simulink model "ES248A_MotAgArbn"  (R2013b)
settings: Solver=FixedStepDiscrete  StartTime=0.0  StopTime=2  FixedStep=0.00005  RelTol=1e-3
undefined symbols (not defined in the file): MAXSTALL_CNT_U08, sigbuilder_block
libraries: simulink x6
settings Model: ModifiedHistory=Rev 008: Updated model to Matlab 2013B, added comments to show requirement linkage  Creator=nz3zln  LastModifiedBy=TZBSJD
settings DataIOCC: SignalLoggingSaveFormat=ModelDataLogs
settings OptimizationCC: InlineParams=on  ExpressionDepthLimit=2147483647
settings DebuggingCC: MultiTaskDSMMsg=none  FcnCallInpInsideContextMsg=UseLocalSettings  StateNameClashWarn=warning
settings GRTTargetCC: CombineOutputUpdateFcns=off  GRTInterface=on

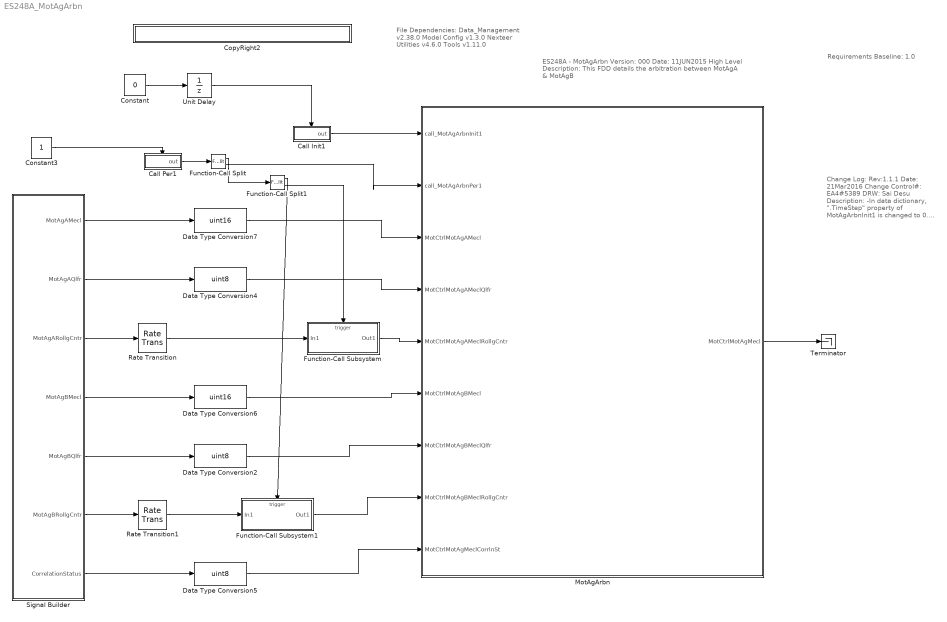
== system ES248A_MotAgArbn ==
  note: ES248A - MotAgArbn
      |
      | Version: 000
      | Date: 11JUN2015
      |
      | High Level Description:
      | This FDD details the arbitration between MotAgA & MotAgB
  note: Change Log:
      | Rev:1.1.1
      | Date: 21Mar2016
      | Change Control#: EA4#5389
      | DRW: Sai Desu
      | Description:
      |  -In data dictionary, ".TimeStep"
      | property of  MotAgArbnInit1 is
      | changed to 0.
      | -In data dictionary, ".Context"
      | property of  MotAgArbnper1 is
      | changed to NonRte.
      |
      | Rev: 1.1.0
      | Date: 13OCT2015
      | Change Control #: EA4#1850
      | DRW: Muragesh Asundi
      | Description:
      | - Init function added
      |
      | Rev: 1.0.0
      | Date: 11JUN2015
      | Change Control #: ICR-TBD
      | DRW: J. Erlenbeck
      | Description:
      | - Initial Release
  note: File Dependencies:
      | Data_Management v2.38.0
      | Model Config v1.3.0
      | Nexteer Utilities v4.6.0
      | Tools v1.11.0
  note: Requirements Baseline: 1.0
  Call Init1 : Subsystem  TreatAsAtomicUnit=on
  Call Per1 : Subsystem  TreatAsAtomicUnit=on
  Constant : Constant  Value=0  OutDataTypeStr=uint8
  Constant3 : Constant  OutDataTypeStr=int8
  CopyRight2 : Subsystem  Description=|  mask(Copyright Information){none=on}
      | Copyright info block.                                               
      |                                                                     
      | Place copyright information at the top of every subsystem in design.
      mask prompts: none "No parameters"
      mask help: Place copyright information at the top of every subsystem in design.
      mask Display:
      | NxtrConf = 'Nexteer Confidential';
      | 
      | sys = bdroot; %handle for the current model ("system")
      | first = get_param(sys,'Created');
      | first = first(end-3:end);  %year is last four digits
      | 
      | last = get_param(sys,'LastModifiedDate');
      | if isempty(last)
      |     last = datestr(now,'yyyy');
      | else
      |     last = last(end-3:end);
      | end
      | 
      | if strcmp(first,last)
      |     fprintf('%s -- Copyright %s Nexteer',NxtrConf,first)
      | else
      |     fprintf('%s -- %s%s- %s Nexteer',NxtrConf,char(169),first,last)
      | end
  Data Type Conversion2 : DataTypeConversion  OutDataTypeStr=uint8  RndMeth=Nearest
  Data Type Conversion4 : DataTypeConversion  OutDataTypeStr=uint8  RndMeth=Nearest
  Data Type Conversion5 : DataTypeConversion  OutDataTypeStr=uint8  RndMeth=Nearest
  Data Type Conversion6 : DataTypeConversion  OutDataTypeStr=uint16  RndMeth=Nearest
  Data Type Conversion7 : DataTypeConversion  OutDataTypeStr=uint16  RndMeth=Nearest
  Function-Call Split : FunctionCallSplit
  Function-Call Split1 : FunctionCallSplit
  Function-Call Subsystem : Subsystem  TreatAsAtomicUnit=on
  Function-Call Subsystem1 : Subsystem  TreatAsAtomicUnit=on
  MotAgArbn : Subsystem
  Rate Transition : RateTransition
  Rate Transition1 : RateTransition
  Signal Builder : Subsystem  Tag=STV Subsys  LoadFcn=sigbuilder_block('load');  StartFcn=sigbuilder_block('start');  StopFcn=sigbuilder_block('stop');  ClipboardFcn=sigbuilder_block('clipboard');  mask(Sigbuilder block){}
      mask help: Simulink:masks:SigbuilderBlock_MD
      mask init:
      | if ~strcmp(get_param(bdroot(gcbh),'SimulationStatus'),'stopped') tuvar = sigbuilder_block('maskInit'); end
      settings: CopyFcn=sigbuilder_block('copy');  DeleteFcn=sigbuilder_block('delete');  ModelCloseFcn=sigbuilder_block('modelClose');  PreSaveFcn=sigbuilder_block('preSave');  PauseFcn=sigbuilder_block('pause');  ContinueFcn=sigbuilder_block('continue');  NameChangeFcn=sigbuilder_block('namechange');  OpenFcn=sigbuilder_block('open',[130.345 51.5172 968.276 555.517 ]);  CloseFcn=sigbuilder_block('close');
      mask Display: plot(0, 0, 100, 100,[2, 2, 32, 32, 2], [68, 8, 8, 68, 68],[32, 2], [38, 38], [32, 19, 2],[53, 60, 44], [32, 17, 17, 2],[16, 16, 31, 31]);txt = getActiveGroup(gcbh);text(2, 100, txt,'verticalAlignment', 'top');
  Terminator : Terminator
  Unit Delay : UnitDelay  InitialCondition=1  SampleTime=-1
  wires:
  Constant3/1 -> Call Per1/Enable
  Call Per1/1(out) -> Function-Call Split/1
  Signal Builder/5(MotAgBQlfr) -> Data Type Conversion2/1
  Signal Builder/4(MotAgBMecl) -> Data Type Conversion6/1
  Signal Builder/3(MotAgARollgCntr) -> Rate Transition/1
  Signal Builder/7(CorrelationStatus) -> Data Type Conversion5/1
  Signal Builder/2(MotAgAQlfr) -> Data Type Conversion4/1
  Signal Builder/1(MotAgAMecl) -> Data Type Conversion7/1
  Data Type Conversion4/1 -> MotAgArbn/4(MotCtrlMotAgAMeclQlfr)
  Data Type Conversion2/1 -> MotAgArbn/7(MotCtrlMotAgBMeclQlfr)
  Data Type Conversion5/1 -> MotAgArbn/9(MotCtrlMotAgMeclCorrlnSt)
  Data Type Conversion6/1 -> MotAgArbn/6(MotCtrlMotAgBMecl)
  Data Type Conversion7/1 -> MotAgArbn/3(MotCtrlMotAgAMecl)
  Function-Call Subsystem/1(Out1) -> MotAgArbn/5(MotCtrlMotAgAMeclRollgCntr)
  Rate Transition/1 -> Function-Call Subsystem/1(In1)
  Signal Builder/6(MotAgBRollgCntr) -> Rate Transition1/1
  Rate Transition1/1 -> Function-Call Subsystem1/1(In1)
  Function-Call Subsystem1/1(Out1) -> MotAgArbn/8(MotCtrlMotAgBMeclRollgCntr)
  Function-Call Split/2 -> MotAgArbn/2(call_MotAgArbnPer1)
  Function-Call Split/1 -> Function-Call Split1/1
  Function-Call Split1/2 -> Function-Call Subsystem/Trigger
  Function-Call Split1/1 -> Function-Call Subsystem1/Trigger
  Call Init1/1(out) -> MotAgArbn/1(call_MotAgArbnInit1)
  Constant/1 -> Unit Delay/1
  Unit Delay/1 -> Call Init1/Enable
  MotAgArbn/1("MotCtrlMotAgMecl ") -> Terminator/1

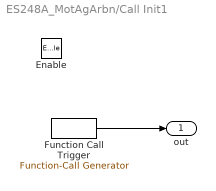
== system ES248A_MotAgArbn/Call Init1 ==
  Enable : EnablePort
  Function Call Trigger : simulink/Ports & Subsystems/Function-Call Generator  RequirementInfo={} %GIDa_03d3be70_2a53_4f3d_90ce_b287f92bdd04  sample_time=0.0005  numberOfIterations=1
  out : Outport
  wires:
  Function Call Trigger/1 -> out/1

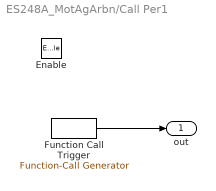
== system ES248A_MotAgArbn/Call Per1 ==
  Enable : EnablePort
  Function Call Trigger : simulink/Ports & Subsystems/Function-Call Generator  RequirementInfo={} %GIDa_6dd05ab1_f91b_4d7a_a0ec_1170d213fa7b  sample_time=0.0005  numberOfIterations=1
  out : Outport
  wires:
  Function Call Trigger/1 -> out/1

== system ES248A_MotAgArbn/CopyRight2 ==

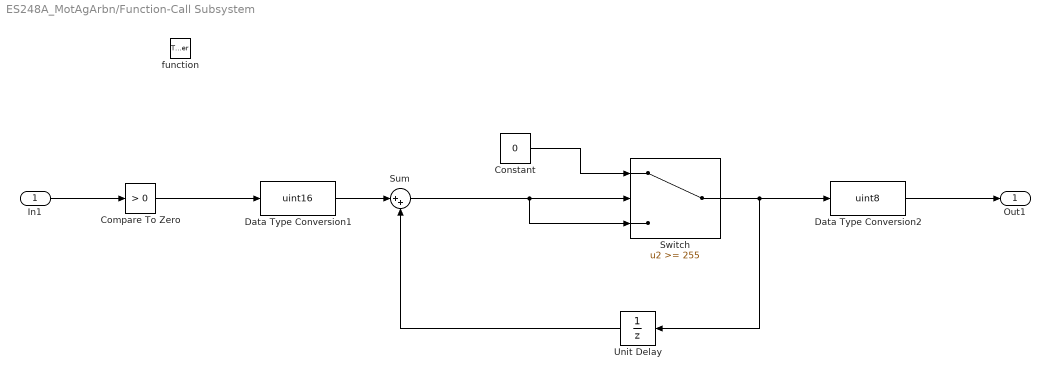
== system ES248A_MotAgArbn/Function-Call Subsystem ==
  In1 : Inport
  function : TriggerPort  TriggerType=function-call
  Compare To Zero : simulink/Logic and Bit Operations/Compare To Zero  relop=>  OutDataTypeStr=uint8
  Constant : Constant  Value=0  OutDataTypeStr=uint16
  Data Type Conversion1 : DataTypeConversion  OutDataTypeStr=uint16  RndMeth=Nearest
  Data Type Conversion2 : DataTypeConversion  OutDataTypeStr=uint8  RndMeth=Nearest
  Sum : Sum  Inputs=|++
  Switch : Switch  Threshold=255
  Unit Delay : UnitDelay  SampleTime=-1
  Out1 : Outport
  wires:
  Constant/1 -> Switch/1
  Sum/1 -> Switch/3, Switch/2
  Data Type Conversion1/1 -> Sum/1
  Switch/1 -> Unit Delay/1, Data Type Conversion2/1
  Data Type Conversion2/1 -> Out1/1
  Unit Delay/1 -> Sum/2
  In1/1 -> Compare To Zero/1
  Compare To Zero/1 -> Data Type Conversion1/1

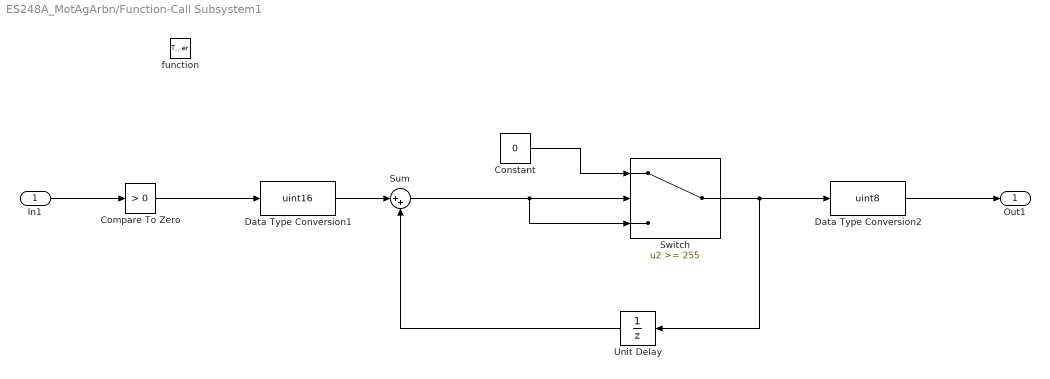
== system ES248A_MotAgArbn/Function-Call Subsystem1 ==
  In1 : Inport
  function : TriggerPort  TriggerType=function-call
  Compare To Zero : simulink/Logic and Bit Operations/Compare To Zero  relop=>  OutDataTypeStr=uint8
  Constant : Constant  Value=0  OutDataTypeStr=uint16
  Data Type Conversion1 : DataTypeConversion  OutDataTypeStr=uint16  RndMeth=Nearest
  Data Type Conversion2 : DataTypeConversion  OutDataTypeStr=uint8  RndMeth=Nearest
  Sum : Sum  Inputs=|++
  Switch : Switch  Threshold=255
  Unit Delay : UnitDelay  SampleTime=-1
  Out1 : Outport
  wires:
  Compare To Zero/1 -> Data Type Conversion1/1
  In1/1 -> Compare To Zero/1
  Unit Delay/1 -> Sum/2
  Data Type Conversion2/1 -> Out1/1
  Switch/1 -> Data Type Conversion2/1, Unit Delay/1
  Data Type Conversion1/1 -> Sum/1
  Sum/1 -> Switch/2, Switch/3
  Constant/1 -> Switch/1

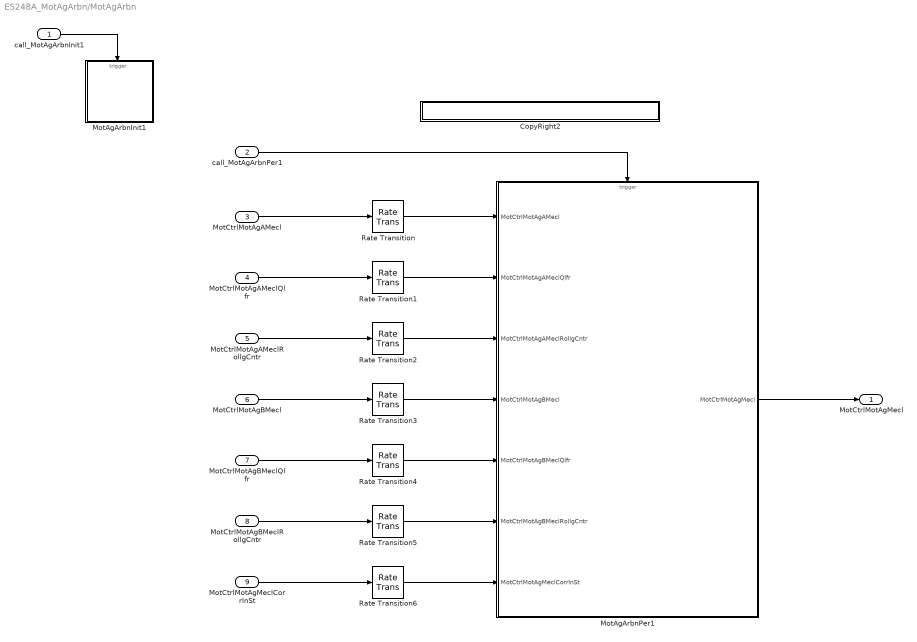
== system ES248A_MotAgArbn/MotAgArbn ==
  call_MotAgArbnInit1 : Inport  RequirementInfo={} %GIDa_2de43c09_82b6_47b9_8e99_1c21e4b82fe2
  call_MotAgArbnPer1 : Inport  RequirementInfo={} %GIDa_468d2479_6710_42ce_bd19_b69834ab6306  Port=2
  MotCtrlMotAgAMecl : Inport  Port=3
  MotCtrlMotAgAMeclQlfr : Inport  Port=4
  MotCtrlMotAgAMeclRollgCntr : Inport  RequirementInfo={} %GIDa_84fb02b3_72b4_4e28_a17f_e99f7297de00  Port=5
  MotCtrlMotAgBMecl : Inport  Port=6
  MotCtrlMotAgBMeclQlfr : Inport  Port=7
  MotCtrlMotAgBMeclRollgCntr : Inport  RequirementInfo={} %GIDa_520df333_aa42_4214_8b7a_2bf2bb8d6174  Port=8
  MotCtrlMotAgMeclCorrlnSt : Inport  Port=9
  CopyRight2 : Subsystem  Description=|  mask(Copyright Information){none=on}
      | Copyright info block.                                               
      |                                                                     
      | Place copyright information at the top of every subsystem in design.
      mask prompts: none "No parameters"
      mask help: Place copyright information at the top of every subsystem in design.
      mask Display:
      | NxtrConf = 'Nexteer Confidential';
      | 
      | sys = bdroot; %handle for the current model ("system")
      | first = get_param(sys,'Created');
      | first = first(end-3:end);  %year is last four digits
      | 
      | last = get_param(sys,'LastModifiedDate');
      | if isempty(last)
      |     last = datestr(now,'yyyy');
      | else
      |     last = last(end-3:end);
      | end
      | 
      | if strcmp(first,last)
      |     fprintf('%s -- Copyright %s Nexteer',NxtrConf,first)
      | else
      |     fprintf('%s -- %s%s- %s Nexteer',NxtrConf,char(169),first,last)
      | end
  MotAgArbnInit1 : Subsystem
  MotAgArbnPer1 : Subsystem  TreatAsAtomicUnit=on
  Rate Transition{,1..6} (7 alike) : RateTransition
  "MotCtrlMotAgMecl " : Outport
  wires:
  call_MotAgArbnPer1/1 -> MotAgArbnPer1/Trigger
  MotAgArbnPer1/1(MotCtrlMotAgMecl) -> "MotCtrlMotAgMecl "/1
  MotCtrlMotAgAMecl/1 -> Rate Transition/1
  MotCtrlMotAgAMeclQlfr/1 -> Rate Transition1/1
  MotCtrlMotAgAMeclRollgCntr/1 -> Rate Transition2/1
  MotCtrlMotAgBMecl/1 -> Rate Transition3/1
  MotCtrlMotAgBMeclQlfr/1 -> Rate Transition4/1
  MotCtrlMotAgBMeclRollgCntr/1 -> Rate Transition5/1
  MotCtrlMotAgMeclCorrlnSt/1 -> Rate Transition6/1
  Rate Transition/1 -> MotAgArbnPer1/1(MotCtrlMotAgAMecl)
  Rate Transition1/1 -> MotAgArbnPer1/2(MotCtrlMotAgAMeclQlfr)
  Rate Transition2/1 -> MotAgArbnPer1/3(MotCtrlMotAgAMeclRollgCntr)
  Rate Transition3/1 -> MotAgArbnPer1/4(MotCtrlMotAgBMecl)
  Rate Transition4/1 -> MotAgArbnPer1/5(MotCtrlMotAgBMeclQlfr)
  Rate Transition6/1 -> MotAgArbnPer1/7(MotCtrlMotAgMeclCorrlnSt)
  Rate Transition5/1 -> MotAgArbnPer1/6(MotCtrlMotAgBMeclRollgCntr)
  call_MotAgArbnInit1/1 -> MotAgArbnInit1/Trigger

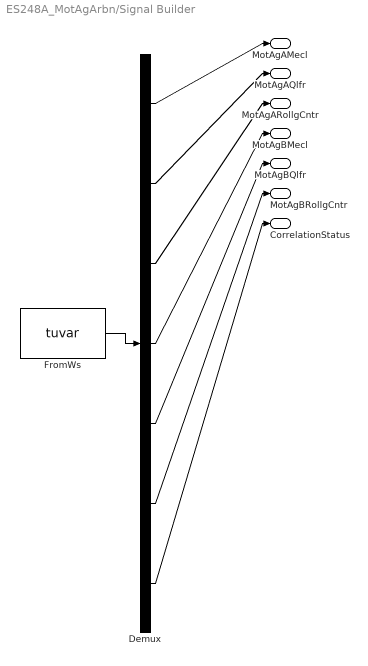
== system ES248A_MotAgArbn/Signal Builder ==
  Demux : Demux  Tag=STV Demux  Outputs=7
  FromWs : FromWorkspace  Tag=STV FromWs  VariableName=tuvar  SampleTime=0
      SigBuilderData=|
      | common.afterFinalStr = 'Extrapolate'
      | common.sampleTime = 0
      | dataSet.timeRange = [0 2]
      | dataSet.name = 'Group 1'
      | sbobj.Groups.Name = 'Group 1'
      | sbobj.Groups.Signals(1).Name = 'MotAgAMecl'
      | sbobj.Groups.Signals(1).XData = [0 0.166666666667 0.166666666667 0.333333333333 0.333333333333 0.5 0.5 0.666666666667 0.666666666667 0.833333333333 0.833333333333 1 1 1.16666666667 1.16666666667 1.33333333333 1.33333333333 1.5 1.5 1.66666666667 1.66666666667 1.83333333333 1.83333333333 2]
      | sbobj.Groups.Signals(1).YData = [0 65534 0 65534 0 65534 0 65534 0 65534 0 65534 0 65534 0 65534 0 65534 0 65534 0 65534 0 65534]
      | sbobj.Groups.Signals(2).Name = 'MotAgAQlfr'
      | sbobj.Groups.Signals(2).XData = [0 0.25 0.25 0.4 0.4 0.71 0.71 0.89 0.89 1.5 2]
      | sbobj.Groups.Signals(2).YData = [1 1 2 2 1 1 2 2 1 1 1]
      | sbobj.Groups.Signals(3).Name = 'MotAgARollgCntr'
      | sbobj.Groups.Signals(3).XData = [0 1.14 1.14 1.3 1.3 1.68 1.68 1.8 1.8 2]
      | sbobj.Groups.Signals(3).YData = [1 1 -1 -1 1 1 -1 -1 1.002 1]
      | sbobj.Groups.Signals(4).Name = 'MotAgBMecl'
      | sbobj.Groups.Signals(4).XData = [0 0.333333333333 0.333333333333 0.666666666667 0.666666666667 1 1 1.33333333333 1.33333333333 1.66666666667 1.66666666667 2]
      | sbobj.Groups.Signals(4).YData = [0 65534 0 65534 0 65534 0 65534 0 65534 0 65534]
      | sbobj.Groups.Signals(5).Name = 'MotAgBQlfr'
      | sbobj.Groups.Signals(5).XData = [0 0.51 0.51 0.6 0.6 0.8 0.8 0.96 0.96 1.5 2]
      | sbobj.Groups.Signals(5).YData = [1 1 2 2 1 1 2 2 1 1 1]
      | sbobj.Groups.Signals(6).Name = 'MotAgBRollgCntr'
      | sbobj.Groups.Signals(6).XData = [0 0.25 1.402 1.402 1.516 1.516 1.746 1.746 1.852 1.852 2]
      | sbobj.Groups.Signals(6).YData = [1 1 1 -1 -1 1 1 -1 -1 1 1]
      | sbobj.Groups.Signals(7).Name = 'CorrelationStatus'
      | sbobj.Groups.Signals(7).XData = [0 0.98 0.98 1.046 1.046 1.914 1.914 1.962 1.962 2]
      | sbobj.Groups.Signals(7).YData = [7 7 5 5 7 7 6 6 7 7]
      | sbobj.Groups.TimeRange = [0 2]
  MotAgAMecl : Outport  Tag=STV Outport
  MotAgAQlfr : Outport  Tag=STV Outport  Port=2
  MotAgARollgCntr : Outport  Tag=STV Outport  Port=3
  MotAgBMecl : Outport  Tag=STV Outport  Port=4
  MotAgBQlfr : Outport  Tag=STV Outport  Port=5
  MotAgBRollgCntr : Outport  Tag=STV Outport  Port=6
  CorrelationStatus : Outport  Tag=STV Outport  Port=7
  wires:
  FromWs/1 -> Demux/1
  Demux/1 -> MotAgAMecl/1
  Demux/2 -> MotAgAQlfr/1
  Demux/3 -> MotAgARollgCntr/1
  Demux/4 -> MotAgBMecl/1
  Demux/5 -> MotAgBQlfr/1
  Demux/6 -> MotAgBRollgCntr/1
  Demux/7 -> CorrelationStatus/1

== system ES248A_MotAgArbn/MotAgArbn/CopyRight2 ==

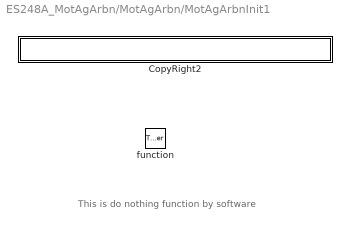
== system ES248A_MotAgArbn/MotAgArbn/MotAgArbnInit1 ==
  note: This is do nothing function by software
  function : TriggerPort  TriggerType=function-call
  CopyRight2 : Subsystem  Description=|  mask(Copyright Information){none=on}
      | Copyright info block.                                               
      |                                                                     
      | Place copyright information at the top of every subsystem in design.
      mask prompts: none "No parameters"
      mask help: Place copyright information at the top of every subsystem in design.
      mask Display:
      | NxtrConf = 'Nexteer Confidential';
      | 
      | sys = bdroot; %handle for the current model ("system")
      | first = get_param(sys,'Created');
      | first = first(end-3:end);  %year is last four digits
      | 
      | last = get_param(sys,'LastModifiedDate');
      | if isempty(last)
      |     last = datestr(now,'yyyy');
      | else
      |     last = last(end-3:end);
      | end
      | 
      | if strcmp(first,last)
      |     fprintf('%s -- Copyright %s Nexteer',NxtrConf,first)
      | else
      |     fprintf('%s -- %s%s- %s Nexteer',NxtrConf,char(169),first,last)
      | end

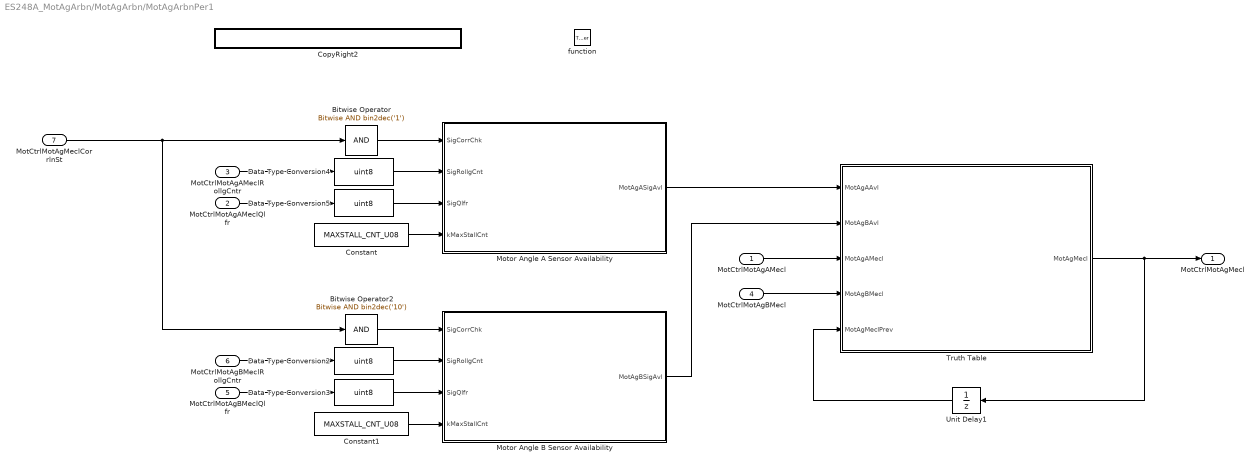
== system ES248A_MotAgArbn/MotAgArbn/MotAgArbnPer1 ==
  MotCtrlMotAgAMecl : Inport
  MotCtrlMotAgAMeclQlfr : Inport  Port=2
  MotCtrlMotAgAMeclRollgCntr : Inport  RequirementInfo={} %GIDa_9d4de4cc_7719_48bf_85c0_912168cfd52f  Port=3
  MotCtrlMotAgBMecl : Inport  Port=4
  MotCtrlMotAgBMeclQlfr : Inport  Port=5
  MotCtrlMotAgBMeclRollgCntr : Inport  RequirementInfo={} %GIDa_f369223d_5d11_4083_be68_0bfa0898a904  Port=6
  MotCtrlMotAgMeclCorrlnSt : Inport  Port=7
  function : TriggerPort  TriggerType=function-call
  Bitwise Operator : simulink/Logic and Bit Operations/Bitwise Operator  logicop=AND  UseBitMask=on  BitMask=bin2dec('1')  BitMaskRealWorld=Stored Integer
  Bitwise Operator2 : simulink/Logic and Bit Operations/Bitwise Operator  logicop=AND  UseBitMask=on  BitMask=bin2dec('10')  BitMaskRealWorld=Stored Integer
  Constant : Constant  Value=MAXSTALL_CNT_U08
  Constant1 : Constant  Value=MAXSTALL_CNT_U08
  CopyRight2 : Subsystem  Description=|  mask(Copyright Information){none=on}
      | Copyright info block.                                               
      |                                                                     
      | Place copyright information at the top of every subsystem in design.
      mask prompts: none "No parameters"
      mask help: Place copyright information at the top of every subsystem in design.
      mask Display:
      | NxtrConf = 'Nexteer Confidential';
      | 
      | sys = bdroot; %handle for the current model ("system")
      | first = get_param(sys,'Created');
      | first = first(end-3:end);  %year is last four digits
      | 
      | last = get_param(sys,'LastModifiedDate');
      | if isempty(last)
      |     last = datestr(now,'yyyy');
      | else
      |     last = last(end-3:end);
      | end
      | 
      | if strcmp(first,last)
      |     fprintf('%s -- Copyright %s Nexteer',NxtrConf,first)
      | else
      |     fprintf('%s -- %s%s- %s Nexteer',NxtrConf,char(169),first,last)
      | end
  Data Type Conversion{2..5} (4 alike) : DataTypeConversion  OutDataTypeStr=uint8  RndMeth=Nearest
  Motor Angle A Sensor Availability : Subsystem  RequirementInfo="{'linktype_rmi_doors' '0000cf49 (/ESG Group/FDD Module Requirements/EA4 Specific/ES248A_MotAgArbn)' '#ES248A_74' 'true' 'REQ:  ES248A_74' '' } %GIDa_a3666822_1018_404e_9f7a_19faaace6442"  TreatAsAtomicUnit=on
  Motor Angle B Sensor Availability : Subsystem  RequirementInfo="{'linktype_rmi_doors' '0000cf49 (/ESG Group/FDD Module Requirements/EA4 Specific/ES248A_MotAgArbn)' '#ES248A_75' 'true' 'REQ:  ES248A_75' '' } %GIDa_28ed2507_8f1c_4e08_96e7_c3d7a5165f80"  TreatAsAtomicUnit=on
  Truth Table : Truth Table  RequirementInfo="{'linktype_rmi_doors' '0000cf49 (/ESG Group/FDD Module Requirements/EA4 Specific/ES248A_MotAgArbn)' '#ES248A_14' 'true' 'REQ:  ES248A_14' '' ; 'linktype_rmi_doors' '0000cf49 (/ESG Group/FDD Module Requirements/EA4 Specific/ES248A_MotAgArbn)' '#ES248A_72' 'true' 'REQ:  ES248A_72' '' ; 'linktype_rmi_doors' '0000cf49 (/ESG Group/FDD Module Requirements/EA4 Specific/ES248A_MotAgArbn)' '#ES248A_73' 'true' 'REQ:  ES248A_73' '' } %GIDa_81496fc9_474b_487e_9fa9_2a6b6ee81132"  TreatAsAtomicUnit=on
  Unit Delay1 : UnitDelay  SampleTime=-1  StateName=MotAgMeclPrev  StateMustResolveToSignalObject=on
      settings: AttributesFormatString=|
      | State Variable:
      | %<StateName>
  MotCtrlMotAgMecl : Outport
  wires:
  MotCtrlMotAgMeclCorrlnSt/1 -> Bitwise Operator2/1, Bitwise Operator/1
  Bitwise Operator/1 -> Motor Angle A Sensor Availability/1(SigCorrChk)
  Constant/1 -> Motor Angle A Sensor Availability/4(kMaxStallCnt)
  MotCtrlMotAgAMeclRollgCntr/1 -> Data Type Conversion4/1
  MotCtrlMotAgAMeclQlfr/1 -> Data Type Conversion5/1
  Data Type Conversion5/1 -> Motor Angle A Sensor Availability/3(SigQlfr)
  Bitwise Operator2/1 -> Motor Angle B Sensor Availability/1(SigCorrChk)
  Constant1/1 -> Motor Angle B Sensor Availability/4(kMaxStallCnt)
  MotCtrlMotAgBMeclRollgCntr/1 -> Data Type Conversion2/1
  MotCtrlMotAgBMeclQlfr/1 -> Data Type Conversion3/1
  Data Type Conversion2/1 -> Motor Angle B Sensor Availability/2(SigRollgCnt)
  Data Type Conversion3/1 -> Motor Angle B Sensor Availability/3(SigQlfr)
  Motor Angle A Sensor Availability/1(MotAgASigAvl) -> Truth Table/1(MotAgAAvl)
  Motor Angle B Sensor Availability/1(MotAgBSigAvl) -> Truth Table/2(MotAgBAvl)
  MotCtrlMotAgAMecl/1 -> Truth Table/3(MotAgAMecl)
  MotCtrlMotAgBMecl/1 -> Truth Table/4(MotAgBMecl)
  Truth Table/1(MotAgMecl) -> Unit Delay1/1, MotCtrlMotAgMecl/1
  Unit Delay1/1 -> Truth Table/5(MotAgMeclPrev)
  Data Type Conversion4/1 -> Motor Angle A Sensor Availability/2(SigRollgCnt)

== system ES248A_MotAgArbn/MotAgArbn/MotAgArbnInit1/CopyRight2 ==

== system ES248A_MotAgArbn/MotAgArbn/MotAgArbnPer1/CopyRight2 ==

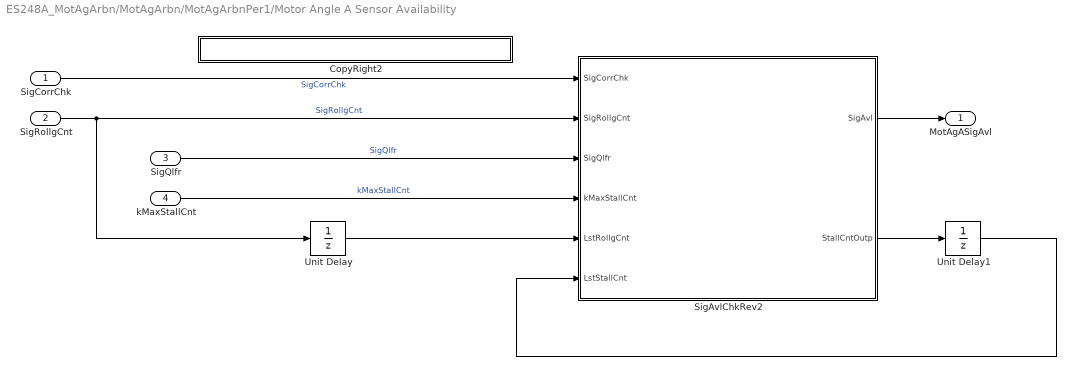
== system ES248A_MotAgArbn/MotAgArbn/MotAgArbnPer1/Motor Angle A Sensor Availability ==
  SigCorrChk : Inport  OutDataTypeStr=uint8
  SigRollgCnt : Inport  Port=2  OutDataTypeStr=uint8
  SigQlfr : Inport  Port=3  OutDataTypeStr=uint8
  kMaxStallCnt : Inport  Port=4  OutDataTypeStr=uint8
  CopyRight2 : Subsystem  Description=|  mask(Copyright Information){none=on}
      | Copyright info block.                                               
      |                                                                     
      | Place copyright information at the top of every subsystem in design.
      mask prompts: none "No parameters"
      mask help: Place copyright information at the top of every subsystem in design.
      mask Display:
      | NxtrConf = 'Nexteer Confidential';
      | 
      | sys = bdroot; %handle for the current model ("system")
      | first = get_param(sys,'Created');
      | first = first(end-3:end);  %year is last four digits
      | 
      | last = get_param(sys,'LastModifiedDate');
      | if isempty(last)
      |     last = datestr(now,'yyyy');
      | else
      |     last = last(end-3:end);
      | end
      | 
      | if strcmp(first,last)
      |     fprintf('%s -- Copyright %s Nexteer',NxtrConf,first)
      | else
      |     fprintf('%s -- %s%s- %s Nexteer',NxtrConf,char(169),first,last)
      | end
  SigAvlChkRev2 : Stateflow chart  TreatAsAtomicUnit=on
  Unit Delay : UnitDelay  SampleTime=-1  StateName=MotAgARollgCntPrev  StateMustResolveToSignalObject=on
      settings: AttributesFormatString=|
      | State Variable:
      | %<StateName>
  Unit Delay1 : UnitDelay  SampleTime=-1  StateName=MotAgAStallCntPrev  StateMustResolveToSignalObject=on
      settings: AttributesFormatString=|
      | State Variable:
      | %<StateName>
  MotAgASigAvl : Outport
  wires:
  SigCorrChk/1 -> SigAvlChkRev2/1(SigCorrChk)  "SigCorrChk"
  SigRollgCnt/1 -> Unit Delay/1, SigAvlChkRev2/2(SigRollgCnt)  "SigRollgCnt"
  SigQlfr/1 -> SigAvlChkRev2/3(SigQlfr)  "SigQlfr"
  kMaxStallCnt/1 -> SigAvlChkRev2/4(kMaxStallCnt)  "kMaxStallCnt"
  Unit Delay/1 -> SigAvlChkRev2/5(LstRollgCnt)
  SigAvlChkRev2/2(StallCntOutp) -> Unit Delay1/1
  Unit Delay1/1 -> SigAvlChkRev2/6(LstStallCnt)
  SigAvlChkRev2/1(SigAvl) -> MotAgASigAvl/1

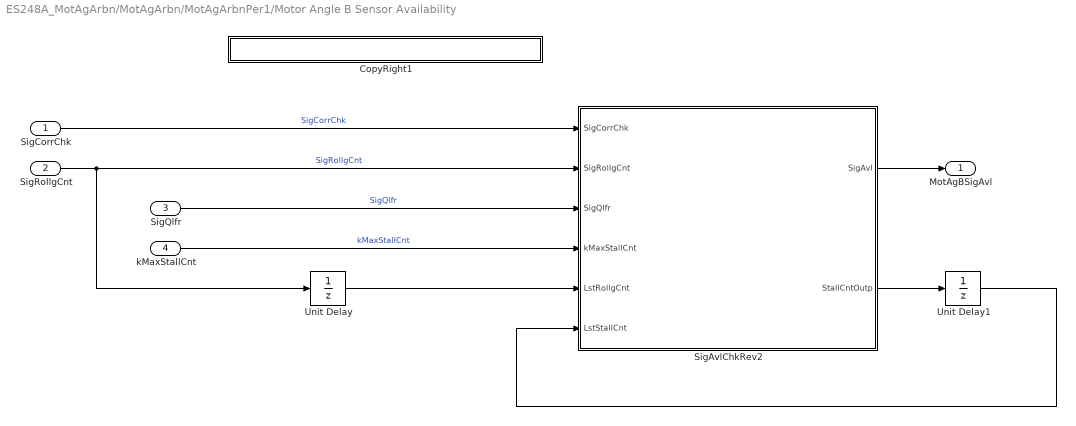
== system ES248A_MotAgArbn/MotAgArbn/MotAgArbnPer1/Motor Angle B Sensor Availability ==
  SigCorrChk : Inport  OutDataTypeStr=uint8
  SigRollgCnt : Inport  Port=2  OutDataTypeStr=uint8
  SigQlfr : Inport  Port=3  OutDataTypeStr=uint8
  kMaxStallCnt : Inport  Port=4  OutDataTypeStr=uint8
  CopyRight1 : Subsystem  Description=|  mask(Copyright Information){none=on}
      | Copyright info block.                                               
      |                                                                     
      | Place copyright information at the top of every subsystem in design.
      mask prompts: none "No parameters"
      mask help: Place copyright information at the top of every subsystem in design.
      mask Display:
      | NxtrConf = 'Nexteer Confidential';
      | 
      | sys = bdroot; %handle for the current model ("system")
      | first = get_param(sys,'Created');
      | first = first(end-3:end);  %year is last four digits
      | 
      | last = get_param(sys,'LastModifiedDate');
      | if isempty(last)
      |     last = datestr(now,'yyyy');
      | else
      |     last = last(end-3:end);
      | end
      | 
      | if strcmp(first,last)
      |     fprintf('%s -- Copyright %s Nexteer',NxtrConf,first)
      | else
      |     fprintf('%s -- %s%s- %s Nexteer',NxtrConf,char(169),first,last)
      | end
  SigAvlChkRev2 : Stateflow chart  TreatAsAtomicUnit=on
  Unit Delay : UnitDelay  SampleTime=-1  StateName=MotAgBRollgCntPrev  StateMustResolveToSignalObject=on
      settings: AttributesFormatString=|
      | State Variable:
      | %<StateName>
  Unit Delay1 : UnitDelay  SampleTime=-1  StateName=MotAgBStallCntPrev  StateMustResolveToSignalObject=on
      settings: AttributesFormatString=|
      | State Variable:
      | %<StateName>
  MotAgBSigAvl : Outport
  wires:
  SigAvlChkRev2/1(SigAvl) -> MotAgBSigAvl/1
  Unit Delay1/1 -> SigAvlChkRev2/6(LstStallCnt)
  SigAvlChkRev2/2(StallCntOutp) -> Unit Delay1/1
  Unit Delay/1 -> SigAvlChkRev2/5(LstRollgCnt)
  kMaxStallCnt/1 -> SigAvlChkRev2/4(kMaxStallCnt)  "kMaxStallCnt"
  SigQlfr/1 -> SigAvlChkRev2/3(SigQlfr)  "SigQlfr"
  SigRollgCnt/1 -> SigAvlChkRev2/2(SigRollgCnt), Unit Delay/1  "SigRollgCnt"
  SigCorrChk/1 -> SigAvlChkRev2/1(SigCorrChk)  "SigCorrChk"

== system ES248A_MotAgArbn/MotAgArbn/MotAgArbnPer1/Motor Angle A Sensor Availability/CopyRight2 ==

== system ES248A_MotAgArbn/MotAgArbn/MotAgArbnPer1/Motor Angle B Sensor Availability/CopyRight1 ==

== matlab function ES248A_MotAgArbn/MotAgArbn/MotAgArbnPer1/Truth Table ==
  data: MotAgAAvl input uint8; MotAgMecl output uint16; MotAgBAvl input uint8; MotAgAMecl input uint16; MotAgBMecl input uint16; MotAgMeclPrev input uint16
function MotAgMecl = fcn(MotAgAAvl, MotAgBAvl, MotAgAMecl, MotAgBMecl, MotAgMeclPrev)

aVarTruthTableCondition_1 = false;
aVarTruthTableCondition_2 = false;


% Motor Angle A is good

aVarTruthTableCondition_1 = logical(MotAgAAvl == 1);

% Motor Angle B is good && Motor Angle A is bad

aVarTruthTableCondition_2 = logical(MotAgBAvl == 1);

if (aVarTruthTableCondition_1)
    aFcnTruthTableAction_1();
elseif (~aVarTruthTableCondition_1 && aVarTruthTableCondition_2)
    aFcnTruthTableAction_2();
else % Default
    aFcnTruthTableAction_3();
end

function aFcnTruthTableAction_1()

% Use Motor Angle A

MotAgMecl = MotAgAMecl;

function aFcnTruthTableAction_2()

% Use Motor Angle B

MotAgMecl = MotAgBMecl;

function aFcnTruthTableAction_3()

% Use Previous Motor Angle

MotAgMecl = MotAgMeclPrev;

== stateflow chart ES248A_MotAgArbn/MotAgArbn/MotAgArbnPer1/Motor Angle B Sensor Availability/SigAvlChkRev2 ==
  note: SigAvl
      | False = 0
      | Pass = 1
  note: SigQlfr
      | 0 = No Result
      | 1 = Pass
      | 2 = Fail
  (default) -> (junction 2)
  (junction 2) -> (junction 4) [order 1] : [SigRollgCnt ==LstRollgCnt]
  (junction 4) -> (junction 7) [order 2] : {
      | StallCntOutp = LstStallCnt +1;
      | }
  (junction 2) -> (junction 3) [order 2]
  (junction 4) -> (junction 7) [order 1] : [LstStallCnt == 255]
      | {
      | StallCntOutp = 255;
      | }
  (junction 3) -> (junction 7) : {
      | StallCntOutp = 0;
      | }
  (junction 7) -> (junction 10)
  (junction 10) -> (junction 12) [order 1] : [StallCntOutp >=kMaxStallCnt]
  (junction 10) -> (junction 14) [order 2]
  (junction 12) -> (junction 17)
  (junction 14) -> (junction 17) [order 2]
  (junction 14) -> (junction 16) [order 1] : [SigQlfr<2 && SigCorrChk>0]
  (junction 17) -> (junction 29) : {
      | SigAvl =0;
      | }
  (junction 16) -> (junction 29) : {
      | SigAvl = 1;
      | }
  data: SigCorrChk input uint8; SigRollgCnt input; SigQlfr input; kMaxStallCnt input; SigAvl output uint8; LstRollgCnt input uint8; LstStallCnt input uint8; StallCntOutp output uint8

== stateflow chart ES248A_MotAgArbn/MotAgArbn/MotAgArbnPer1/Motor Angle A Sensor Availability/SigAvlChkRev2 ==
  note: SigAvl
      | False = 0
      | Pass = 1
  note: SigQlfr
      | 0 = No Result
      | 1 = Pass
      | 2 = Fail
  (default) -> (junction 2)
  (junction 2) -> (junction 4) [order 1] : [SigRollgCnt ==LstRollgCnt]
  (junction 4) -> (junction 7) [order 2] : {
      | StallCntOutp = LstStallCnt +1;
      | }
  (junction 2) -> (junction 3) [order 2]
  (junction 4) -> (junction 7) [order 1] : [LstStallCnt == 255]
      | {
      | StallCntOutp = 255;
      | }
  (junction 3) -> (junction 7) : {
      | StallCntOutp = 0;
      | }
  (junction 7) -> (junction 10)
  (junction 10) -> (junction 12) [order 1] : [StallCntOutp >=kMaxStallCnt]
  (junction 10) -> (junction 14) [order 2]
  (junction 12) -> (junction 17)
  (junction 14) -> (junction 17) [order 2]
  (junction 14) -> (junction 16) [order 1] : [SigQlfr<2 && SigCorrChk>0]
  (junction 17) -> (junction 29) : {
      | SigAvl =0;
      | }
  (junction 16) -> (junction 29) : {
      | SigAvl = 1;
      | }
  data: SigCorrChk input uint8; SigRollgCnt input; SigQlfr input; kMaxStallCnt input; SigAvl output uint8; LstRollgCnt input uint8; LstStallCnt input uint8; StallCntOutp output uint8
